simulink model "bai1"  (R2015a)
settings: Solver=ode45  StartTime=0.0  StopTime=100  RelTol=1e-3
settings Model: Creator=Win 10  LastModifiedBy=Win 10

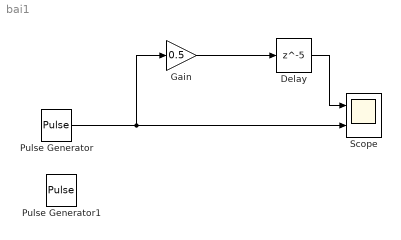
== system bai1 ==
  Delay : Delay  DelayLength=5  SampleTime=1
  Gain : Gain  Gain=0.5
  Pulse Generator : DiscretePulseGenerator  PulseType=Time based  Period=10  PulseWidth=5
  Pulse Generator1 : DiscretePulseGenerator  PulseType=Time based  Period=10  PulseWidth=5
  Scope : Scope  NumInputPorts=2
      settings: YMin=-5~-5  YMax=5~5
  wires:
  Pulse Generator/1 -> Gain/1, Scope/2
  Gain/1 -> Delay/1
  Delay/1 -> Scope/1
